simulink model "SimulationModel"  (R2020a)
settings: Solver=VariableStepAuto  StartTime=0.0  StopTime=100  RelTol=1e-3
values from neighbouring files (symbols this model uses):
  Amp_denom = 5000    [Simulation_parameters.m]
  Amp_num = 5000    [Simulation_parameters.m]
  B = 0.0007    [Simulation_parameters.m]
  J = 9.545e-6    (= 9.545e-06)    [Simulation_parameters.m]
  Km = 35.6e-3    (= 0.0356)    [Simulation_parameters.m]
  Kp = 50    [Simulation_parameters.m]
  Kv = 1./(268./60*2*pi)    (= 0.0356317036773)    [Simulation_parameters.m]
  L = 1.320e-3    (= 0.00132)    [Simulation_parameters.m]
  R = 22.8    [Simulation_parameters.m]
settings Model: Creator=nisch  LastModifiedBy=nisch

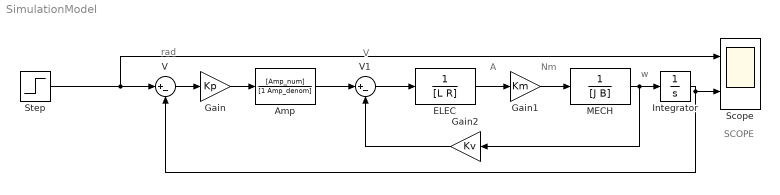
== system SimulationModel ==
  note: SCOPE
  note: w
  note: A
  note: V
  note: rad
  note: Nm
  Amp : TransferFcn  Numerator=[Amp_num]  Denominator=[1 Amp_denom]
  ELEC : TransferFcn  Denominator=[L R]
  Gain : Gain  Gain=Kp
  Gain1 : Gain  Gain=Km
  Gain2 : Gain  Gain=Kv
  Integrator : Integrator
  MECH : TransferFcn  Denominator=[J B]
  Scope : Scope  NumInputPorts=2
  Step : Step  After=pi/2  SampleTime=0
  V : Sum  Inputs=|+-
  V1 : Sum  Inputs=|+-
  wires:
  ELEC/1 -> Gain1/1
  V/1 -> Gain/1
  Step/1 -> Scope/1, V/1
  Gain1/1 -> MECH/1
  MECH/1 -> Gain2/1, Integrator/1
  Integrator/1 -> V/2, Scope/2
  Gain/1 -> Amp/1
  Amp/1 -> V1/1
  V1/1 -> ELEC/1
  Gain2/1 -> V1/2
